simulink model "model_robot"  (Simulink 7.9)
settings: Solver=ode45  StartTime=0.0  StopTime=10.0  RelTol=1e-3
values from neighbouring files (symbols this model uses):
  sx_d = [time sx_d]    [WPG_results.m]    (also in WPG_sim.m; control_layer_zmp_com_init.m = [time sx_d_y]; control_layer_zmp_com_init_2.m = [time sx_d_x])
  w = wpg_param.w    [WPG_results.m]    (also in WPG_results_10.m; WPG_results_2.m; WPG_results_3.m; WPG_results_4.m)
  x_d = [time x_d]    [WPG_results.m]    (also in WPG_sim.m; control_layer_zmp_com_init.m = [time x_d_y]; control_layer_zmp_com_init_2.m = [time x_d_x])
settings Model: Creator=pajon  LastModifiedBy=pajon

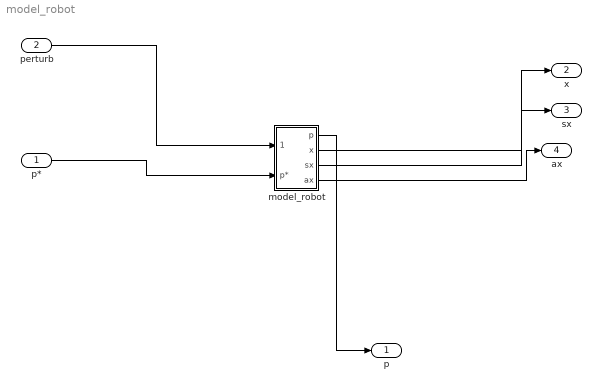
== system model_robot ==
  p* : Inport
  perturb : Inport  Port=2
  model_robot : Subsystem
  p : Outport
  x : Outport  Port=2
  sx : Outport  Port=3
  ax : Outport  Port=4
  wires:
  perturb/1 -> model_robot/1(perturb)
  model_robot/1(p) -> p/1
  model_robot/2(x) -> x/1
  model_robot/3(sx) -> sx/1
  model_robot/4(ax) -> ax/1
  p*/1 -> model_robot/2(p*)

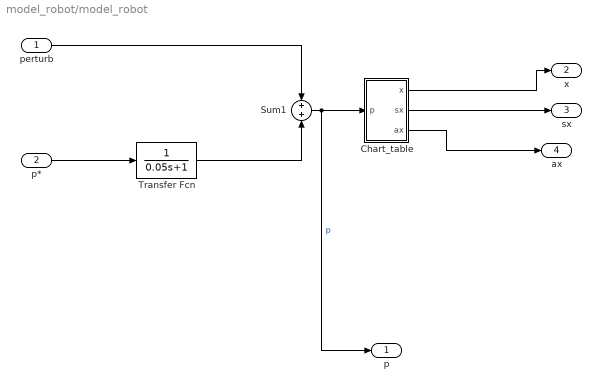
== system model_robot/model_robot ==
  perturb : Inport
  p* : Inport  Port=2
  Chart_table : Subsystem
  Sum1 : Sum
  Transfer Fcn : TransferFcn  Denominator=[0.05 1]
  p : Outport
  x : Outport  Port=2
  sx : Outport  Port=3
  ax : Outport  Port=4
  wires:
  perturb/1 -> Sum1/1
  p*/1 -> Transfer Fcn/1
  Chart_table/1(x) -> x/1
  Chart_table/2(sx) -> sx/1
  Chart_table/3(ax) -> ax/1
  Transfer Fcn/1 -> Sum1/2
  Sum1/1 -> Chart_table/1(p), p/1  "p"

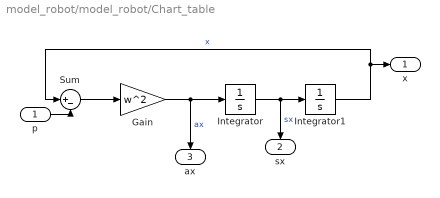
== system model_robot/model_robot/Chart_table ==
  p : Inport
  Gain : Gain  Gain=w^2
  Integrator : Integrator  InitialCondition=sx_d(1,2)
  Integrator1 : Integrator  InitialCondition=x_d(1,2)
  Sum : Sum  Inputs=|+-
  x : Outport
  sx : Outport  Port=2
  ax : Outport  Port=3
  wires:
  Integrator/1 -> Integrator1/1, sx/1  "sx"
  Integrator1/1 -> Sum/1, x/1  "x"
  Gain/1 -> Integrator/1, ax/1  "ax"
  Sum/1 -> Gain/1
  p/1 -> Sum/2
